simulink model "grafica2_practica1_ejer2"  (R2021b)
settings: Solver=VariableStepAuto  StartTime=0.0  StopTime=10.0  RelTol=1e-3
settings Model: Creator=andrea  LastModifiedBy=david

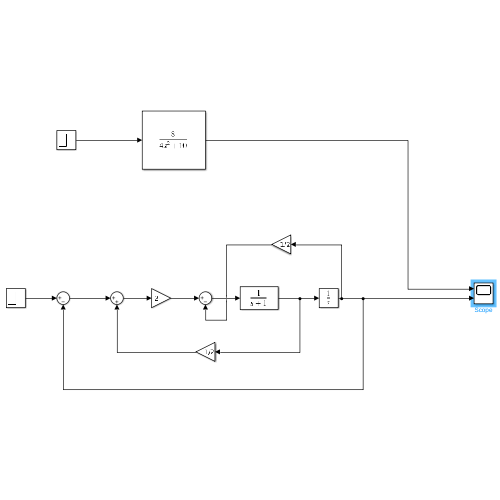
[thumbnail: Simulink's stored preview of the top-level diagram]
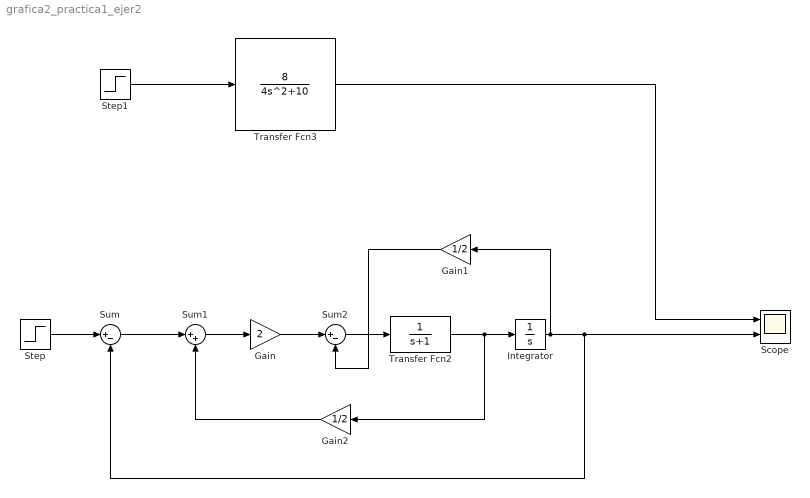
== system grafica2_practica1_ejer2 ==
  Gain : Gain  Gain=2
  Gain1 : Gain  Gain=1/2
  Gain2 : Gain  Gain=1/2
  Integrator : Integrator
  Scope : Scope  NumInputPorts=2
  Step : Step  SampleTime=0
  Step1 : Step  SampleTime=0
  Sum : Sum  Inputs=|+-
  Sum1 : Sum  Inputs=|++
  Sum2 : Sum  Inputs=|+-
  Transfer Fcn2 : TransferFcn  Denominator=[1 1]
  Transfer Fcn3 : TransferFcn  Numerator=[8]  Denominator=[4 0 10]
  wires:
  Step/1 -> Sum/1
  Sum/1 -> Sum1/1
  Sum1/1 -> Gain/1
  Gain/1 -> Sum2/1
  Sum2/1 -> Transfer Fcn2/1
  Transfer Fcn2/1 -> Gain2/1, Integrator/1
  Integrator/1 -> Sum/2, Scope/2, Gain1/1
  Gain1/1 -> Sum2/2
  Gain2/1 -> Sum1/2
  Step1/1 -> Transfer Fcn3/1
  Transfer Fcn3/1 -> Scope/1
